simulink model "manufacturing_final"  (R2016a)
settings: Solver=FixedStepAuto  StartTime=0.0  StopTime=40  FixedStep=0.1  RelTol=1e-3
settings Model: Creator=yshun  LastModifiedBy=yshun

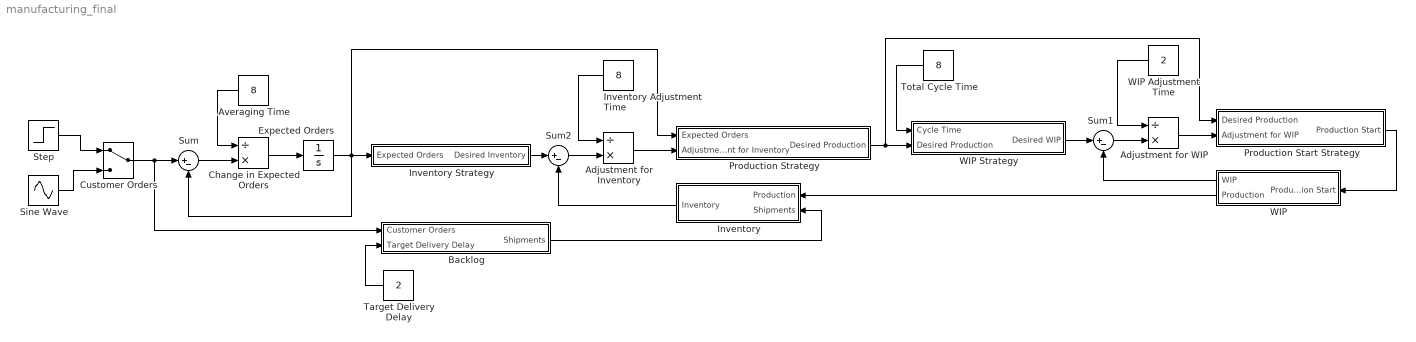
== system manufacturing_final ==
  Adjustment for Inventory : Product  Inputs=/*
  Adjustment for WIP : Product  Inputs=/*
  Averaging Time : Constant  Value=8
  Backlog : Subsystem
  Change in Expected Orders : Product  Inputs=/*
  Customer Orders : ManualSwitch
  Expected Orders : Integrator  InitialCondition=10000
  Inventory : Subsystem
  Inventory Adjustment Time : Constant  Value=8
  Inventory Strategy : Subsystem
  Production Start Strategy : Subsystem
  Production Strategy : Subsystem
  Sine Wave : Sin  SampleTime=0
  Step : Step  Time=5  Before=10000  After=12000  SampleTime=0
  Sum : Sum  Inputs=|+-
  Sum1 : Sum  Inputs=|+-
  Sum2 : Sum  Inputs=|+-
  Target Delivery Delay : Constant  Value=2
  Total Cycle Time : Constant  Value=8
  WIP : Subsystem
  WIP Adjustment Time : Constant  Value=2
  WIP Strategy : Subsystem
  wires:
  Sum/1 -> Change in Expected Orders/2
  Expected Orders/1 -> Sum/2, Production Strategy/1(Expected Orders), Inventory Strategy/1(Expected Orders)
  Inventory Strategy/1(Desired Inventory) -> Sum2/1
  Change in Expected Orders/1 -> Expected Orders/1
  Averaging Time/1 -> Change in Expected Orders/1
  Sum2/1 -> Adjustment for Inventory/2
  Adjustment for Inventory/1 -> Production Strategy/2(Adjustment for Inventory)
  Inventory Adjustment Time/1 -> Adjustment for Inventory/1
  Sum1/1 -> Adjustment for WIP/2
  WIP Adjustment Time/1 -> Adjustment for WIP/1
  WIP Strategy/1(Desired WIP) -> Sum1/1
  Production Strategy/1(Desired Production) -> Production Start Strategy/1("Desired Production "), WIP Strategy/2(Desired Production)
  Adjustment for WIP/1 -> Production Start Strategy/2(Adjustment for WIP)
  Production Start Strategy/1(Production Start) -> WIP/1(Production Start)
  WIP/2(Production) -> Inventory/1(Production)
  Inventory/1(Inventory) -> Sum2/2
  Total Cycle Time/1 -> WIP Strategy/1(Cycle Time)
  WIP/1(WIP) -> Sum1/2
  Customer Orders/1 -> Backlog/1(Customer Orders), Sum/1
  Step/1 -> Customer Orders/1
  Sine Wave/1 -> Customer Orders/2
  Backlog/1(Shipments) -> Inventory/2(Shipments)
  Target Delivery Delay/1 -> Backlog/2(Target Delivery Delay)

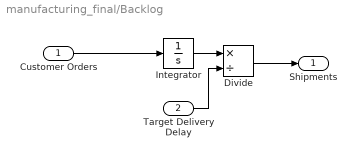
== system manufacturing_final/Backlog ==
  Customer Orders : Inport
  Target Delivery Delay : Inport  Port=2
  Divide : Product  Inputs=*/
  Integrator : Integrator  InitialCondition=20000
  Shipments : Outport
  wires:
  Customer Orders/1 -> Integrator/1
  Integrator/1 -> Divide/1
  Target Delivery Delay/1 -> Divide/2
  Divide/1 -> Shipments/1

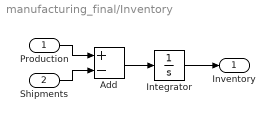
== system manufacturing_final/Inventory ==
  Production : Inport
  Shipments : Inport  Port=2
  Add : Sum  Inputs=+-
  Integrator : Integrator  InitialCondition=40000
  Inventory : Outport
  wires:
  Production/1 -> Add/1
  Shipments/1 -> Add/2
  Add/1 -> Integrator/1
  Integrator/1 -> Inventory/1

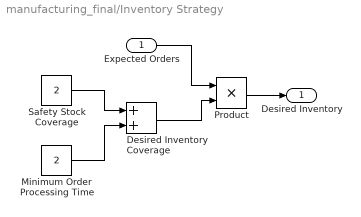
== system manufacturing_final/Inventory Strategy ==
  Expected Orders : Inport
  Desired Inventory Coverage : Sum
  Minimum Order Processing Time : Constant  Value=2
  Product : Product
  Safety Stock Coverage : Constant  Value=2
  Desired Inventory : Outport
  wires:
  Safety Stock Coverage/1 -> Desired Inventory Coverage/1
  Minimum Order Processing Time/1 -> Desired Inventory Coverage/2
  Expected Orders/1 -> Product/1
  Desired Inventory Coverage/1 -> Product/2
  Product/1 -> Desired Inventory/1

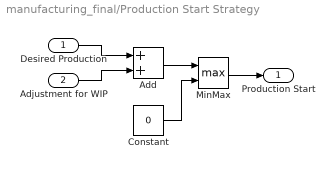
== system manufacturing_final/Production Start Strategy ==
  "Desired Production " : Inport
  Adjustment for WIP : Inport  Port=2
  Add : Sum
  Constant : Constant  Value=0
  MinMax : MinMax  Function=max  Inputs=2
  Production Start : Outport
  wires:
  "Desired Production "/1 -> Add/1
  Adjustment for WIP/1 -> Add/2
  Add/1 -> MinMax/1
  Constant/1 -> MinMax/2
  MinMax/1 -> Production Start/1

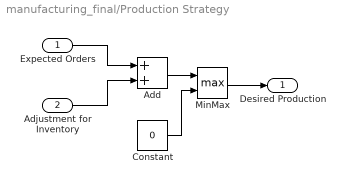
== system manufacturing_final/Production Strategy ==
  Expected Orders : Inport
  Adjustment for Inventory : Inport  Port=2
  Add : Sum
  Constant : Constant  Value=0
  MinMax : MinMax  Function=max  Inputs=2
  Desired Production : Outport
  wires:
  Expected Orders/1 -> Add/1
  Adjustment for Inventory/1 -> Add/2
  Add/1 -> MinMax/1
  Constant/1 -> MinMax/2
  MinMax/1 -> Desired Production/1

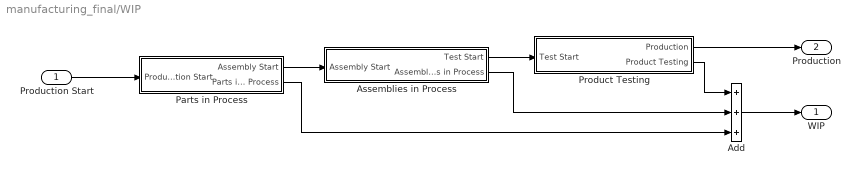
== system manufacturing_final/WIP ==
  Production Start : Inport
  Add : Sum  Inputs=+++
  Assemblies in Process : Subsystem
  Parts in Process : Subsystem
  Product Testing : Subsystem
  WIP : Outport
  Production : Outport  Port=2
  wires:
  Production Start/1 -> Parts in Process/1(Production Start)
  Parts in Process/1(Assembly Start) -> Assemblies in Process/1(Assembly Start)
  Add/1 -> WIP/1
  Parts in Process/2(Parts in Process) -> Add/3
  Assemblies in Process/2(Assemblies in Process) -> Add/2
  Assemblies in Process/1(Test Start) -> Product Testing/1(Test Start)
  Product Testing/2(Product Testing) -> Add/1
  Product Testing/1(Production) -> Production/1

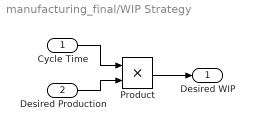
== system manufacturing_final/WIP Strategy ==
  Cycle Time : Inport
  Desired Production : Inport  Port=2
  Product : Product
  Desired WIP : Outport
  wires:
  Desired Production/1 -> Product/2
  Product/1 -> Desired WIP/1
  Cycle Time/1 -> Product/1

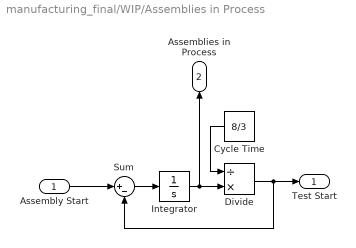
== system manufacturing_final/WIP/Assemblies in Process ==
  Assembly Start : Inport
  Cycle Time : Constant  Value=8/3
  Divide : Product  Inputs=/*
  Integrator : Integrator  InitialCondition=80000/3
  Sum : Sum  Inputs=|+-
  Test Start : Outport
  Assemblies in Process : Outport  Port=2
  wires:
  Assembly Start/1 -> Sum/1
  Sum/1 -> Integrator/1
  Integrator/1 -> Assemblies in Process/1, Divide/2
  Cycle Time/1 -> Divide/1
  Divide/1 -> Test Start/1, Sum/2

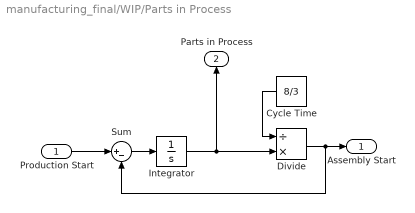
== system manufacturing_final/WIP/Parts in Process ==
  Production Start : Inport
  Cycle Time : Constant  Value=8/3
  Divide : Product  Inputs=/*
  Integrator : Integrator  InitialCondition=80000/3
  Sum : Sum  Inputs=|+-
  Assembly Start : Outport
  Parts in Process : Outport  Port=2
  wires:
  Production Start/1 -> Sum/1
  Sum/1 -> Integrator/1
  Integrator/1 -> Divide/2, Parts in Process/1
  Cycle Time/1 -> Divide/1
  Divide/1 -> Sum/2, Assembly Start/1

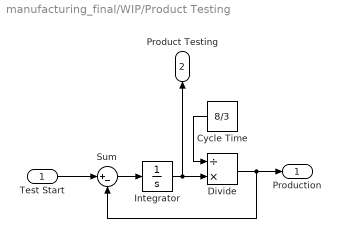
== system manufacturing_final/WIP/Product Testing ==
  Test Start : Inport
  Cycle Time : Constant  Value=8/3
  Divide : Product  Inputs=/*
  Integrator : Integrator  InitialCondition=80000/3
  Sum : Sum  Inputs=|+-
  Production : Outport
  Product Testing : Outport  Port=2
  wires:
  Test Start/1 -> Sum/1
  Sum/1 -> Integrator/1
  Integrator/1 -> Product Testing/1, Divide/2
  Cycle Time/1 -> Divide/1
  Divide/1 -> Production/1, Sum/2
